simulink model "carlaControlInterface"  (R2026a)
settings: Solver=VariableStepAuto
undefined symbols (not defined in the file or in its folder): carlaConfig
settings Model: Creator=ADITYA  LastModifiedBy=ADITYA

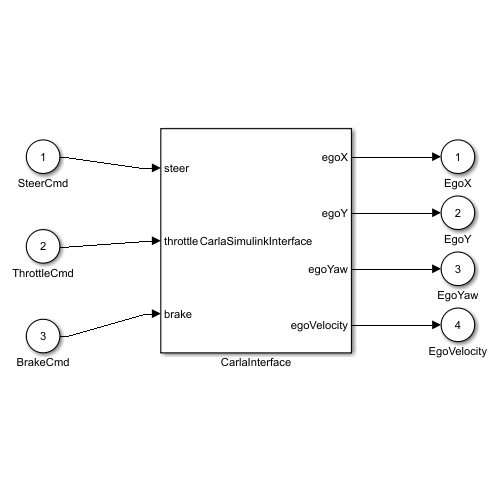
[thumbnail: Simulink's stored preview of the top-level diagram]
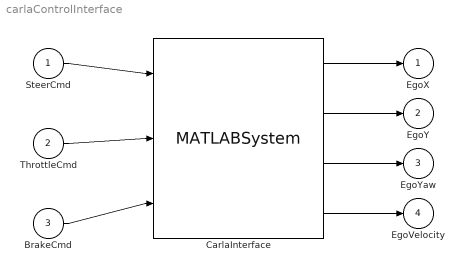
== system carlaControlInterface ==
  SteerCmd : Inport
  ThrottleCmd : Inport  Port=2
  BrakeCmd : Inport  Port=3
  CarlaInterface : MATLABSystem  System=CarlaSimulinkInterface  CarlaCfg=carlaConfig()  SimulateUsing=Interpreted execution
      mask Type: CarlaSimulinkInterface
  EgoX : Outport
  EgoY : Outport  Port=2
  EgoYaw : Outport  Port=3
  EgoVelocity : Outport  Port=4
  wires:
  SteerCmd/1 -> CarlaInterface/1
  ThrottleCmd/1 -> CarlaInterface/2
  BrakeCmd/1 -> CarlaInterface/3
  CarlaInterface/1 -> EgoX/1
  CarlaInterface/2 -> EgoY/1
  CarlaInterface/3 -> EgoYaw/1
  CarlaInterface/4 -> EgoVelocity/1
